simulink model "Microgrid_W"  (R2020a)
settings: Solver=ode15s  StartTime=0  StopTime=1440*1  MaxStep=1  RelTol=1e-3
libraries: simulink x4214, powerlib x685, simulink_extras x28, Microgrid_Library x18, powerlib_meascontrol x12
(part 4 of 48)

== system Microgrid_W/House 2 W3/Light 4 ==
  Add : Sum  Inputs=+++++++
  D1 : Subsystem
  D2 : Subsystem
  D3 : Subsystem
  D4 : Subsystem
  D5 : Subsystem
  D6 : Subsystem
  D7 : Subsystem
  Ground : powerlib/Elements/Ground  LConnTagsString=a
  Ideal Switch : powerlib/Power Electronics/Ideal Switch  Ron=V^2/(K_L3_W+0.000001)  Lon=0  IC=0  Rs=1e5  Cs=inf  Measurements=on
  + : PMIOPort  Side=Left
  wires:
  D7/1(Out1) -> Add/7
  D6/1(Out1) -> Add/6
  D5/1(Out1) -> Add/5
  D4/1(Out1) -> Add/4
  D3/1(Out1) -> Add/3
  D2/1(Out1) -> Add/2
  D1/1(Out1) -> Add/1
  Add/1 -> Ideal Switch/1
  connections:
  Ground/LConn1 -- Ideal Switch/LConn1
  +/RConn1 -- Ideal Switch/RConn1

== system Microgrid_W/House 2 W3/Light 5 ==
  Add : Sum  Inputs=+++++++
  D1 : Subsystem
  D2 : Subsystem
  D3 : Subsystem
  D4 : Subsystem
  D5 : Subsystem
  D6 : Subsystem
  D7 : Subsystem
  Ground : powerlib/Elements/Ground  LConnTagsString=a
  Ideal Switch : powerlib/Power Electronics/Ideal Switch  Ron=V^2/(K_L4_W+0.000001)  Lon=0  IC=0  Rs=1e5  Cs=inf  Measurements=on
  + : PMIOPort  Side=Left
  wires:
  D7/1(Out1) -> Add/7
  D6/1(Out1) -> Add/6
  D5/1(Out1) -> Add/5
  D4/1(Out1) -> Add/4
  D3/1(Out1) -> Add/3
  D2/1(Out1) -> Add/2
  D1/1(Out1) -> Add/1
  Add/1 -> Ideal Switch/1
  connections:
  Ground/LConn1 -- Ideal Switch/LConn1
  +/RConn1 -- Ideal Switch/RConn1

== system Microgrid_W/House 2 W3/Light 6 ==
  Add : Sum  Inputs=+++++++
  D1 : Subsystem
  D2 : Subsystem
  D3 : Subsystem
  D4 : Subsystem
  D5 : Subsystem
  D6 : Subsystem
  D7 : Subsystem
  Ground : powerlib/Elements/Ground  LConnTagsString=a
  Ideal Switch : powerlib/Power Electronics/Ideal Switch  Ron=V^2/(K_L5_W+0.000001)  Lon=0  IC=0  Rs=1e5  Cs=inf  Measurements=on
  + : PMIOPort  Side=Left
  wires:
  D1/1(Out1) -> Add/1
  D2/1(Out1) -> Add/2
  D3/1(Out1) -> Add/3
  D4/1(Out1) -> Add/4
  D5/1(Out1) -> Add/5
  D6/1(Out1) -> Add/6
  D7/1(Out1) -> Add/7
  Add/1 -> Ideal Switch/1
  connections:
  Ground/LConn1 -- Ideal Switch/LConn1
  +/RConn1 -- Ideal Switch/RConn1

== system Microgrid_W/House 2 W3/Light 7 ==
  Add : Sum  Inputs=+++++++
  D1 : Subsystem
  D2 : Subsystem
  D3 : Subsystem
  D4 : Subsystem
  D5 : Subsystem
  D6 : Subsystem
  D7 : Subsystem
  Ground : powerlib/Elements/Ground  LConnTagsString=a
  Ideal Switch : powerlib/Power Electronics/Ideal Switch  Ron=V^2/(K_L6_W+0.000001)  Lon=0  IC=0  Rs=1e5  Cs=inf  Measurements=on
  + : PMIOPort  Side=Left
  wires:
  D7/1(Out1) -> Add/7
  D6/1(Out1) -> Add/6
  D5/1(Out1) -> Add/5
  D4/1(Out1) -> Add/4
  D3/1(Out1) -> Add/3
  D2/1(Out1) -> Add/2
  D1/1(Out1) -> Add/1
  Add/1 -> Ideal Switch/1
  connections:
  Ground/LConn1 -- Ideal Switch/LConn1
  +/RConn1 -- Ideal Switch/RConn1

== system Microgrid_W/House 2 W3/Oven ==
  Add : Sum  Inputs=+++++++
  D1 : Subsystem
  D2 : Subsystem
  D3 : Subsystem
  D4 : Subsystem
  D5 : Subsystem
  D6 : Subsystem
  D7 : Subsystem
  Ground : powerlib/Elements/Ground  LConnTagsString=a
  Ideal Switch : powerlib/Power Electronics/Ideal Switch  Ron=V^2/(825*N_Elements+0.000001)  Lon=0  IC=0  Rs=1e5  Cs=inf  Measurements=on
  + : PMIOPort  Side=Left
  wires:
  D7/1(Out1) -> Add/7
  D6/1(Out1) -> Add/6
  D5/1(Out1) -> Add/5
  D4/1(Out1) -> Add/4
  D3/1(Out1) -> Add/3
  D2/1(Out1) -> Add/2
  D1/1(Out1) -> Add/1
  Add/1 -> Ideal Switch/1
  connections:
  +/RConn1 -- Ideal Switch/RConn1
  Ground/LConn1 -- Ideal Switch/LConn1

== system Microgrid_W/House 2 W3/Phone_Charger ==
  Add : Sum  Inputs=+++++++
  Add1 : Sum  Inputs=+++++++
  Add2 : Sum  Inputs=+++++++
  D1 : Subsystem
  D10 : Subsystem
  D11 : Subsystem
  D12 : Subsystem
  D13 : Subsystem
  D14 : Subsystem
  D15 : Subsystem
  D16 : Subsystem
  D17 : Subsystem
  D18 : Subsystem
  D19 : Subsystem
  D2 : Subsystem
  D20 : Subsystem
  D21 : Subsystem
  D3 : Subsystem
  D4 : Subsystem
  D5 : Subsystem
  D6 : Subsystem
  D7 : Subsystem
  D8 : Subsystem
  D9 : Subsystem
  Ground : powerlib/Elements/Ground  LConnTagsString=a
  Ideal Switch : powerlib/Power Electronics/Ideal Switch  Ron=V^2/(Phone_C_1_W+0.000001)  Lon=0  IC=0  Rs=1e5  Cs=inf  Measurements=on
  Ideal Switch1 : powerlib/Power Electronics/Ideal Switch  Ron=V^2/(Phone_C_2_W+0.000001)  Lon=0  IC=0  Rs=1e5  Cs=inf  Measurements=on
  Ideal Switch2 : powerlib/Power Electronics/Ideal Switch  Ron=V^2/(Phone_C_3_W+0.000001)  Lon=0  IC=0  Rs=1e5  Cs=inf  Measurements=on
  + : PMIOPort  Side=Left
  +1 : PMIOPort  Port=2  Side=Right
  +2 : PMIOPort  Port=3  Side=Left
  wires:
  D1/1(Out1) -> Add/1
  D2/1(Out1) -> Add/2
  D3/1(Out1) -> Add/3
  D4/1(Out1) -> Add/4
  D5/1(Out1) -> Add/5
  D6/1(Out1) -> Add/6
  D7/1(Out1) -> Add/7
  D8/1(Out1) -> Add1/1
  D9/1(Out1) -> Add1/2
  D10/1(Out1) -> Add1/3
  D11/1(Out1) -> Add1/4
  D12/1(Out1) -> Add1/5
  D13/1(Out1) -> Add1/6
  D14/1(Out1) -> Add1/7
  D20/1(Out1) -> Add2/1
  D15/1(Out1) -> Add2/2
  D16/1(Out1) -> Add2/3
  D17/1(Out1) -> Add2/4
  D18/1(Out1) -> Add2/5
  D19/1(Out1) -> Add2/6
  D21/1(Out1) -> Add2/7
  Add/1 -> Ideal Switch/1
  Add1/1 -> Ideal Switch1/1
  Add2/1 -> Ideal Switch2/1
  connections:
  Ground/LConn1 -- Ideal Switch2/LConn1 -- Ideal Switch1/LConn1 -- Ideal Switch/LConn1
  +/RConn1 -- Ideal Switch/RConn1
  +1/RConn1 -- Ideal Switch1/RConn1
  +2/RConn1 -- Ideal Switch2/RConn1

== system Microgrid_W/House 2 W3/Refrigerator ==
  Current Measurement : powerlib/Measurements/Current Measurement  PhasorSimulation=off  OutputType=Complex  PSBequivalent=0
  Ground : powerlib/Elements/Ground  LConnTagsString=a
  Ideal Switch : powerlib/Power Electronics/Ideal Switch  Ron=0.01  Lon=0  IC=0  Rs=1e5  Cs=inf  Measurements=on
  Ideal Switch1 : powerlib/Power Electronics/Ideal Switch  Ron=0.01  Lon=0  IC=0  Rs=1e5  Cs=inf  Measurements=on
  Monostable : powerlib_meascontrol/Logic/Monostable  EdgeDetect=Rising  PulseDuration=0.1*(60/t)  ic=0  Ts=0
      settings: SourceProductBaseCode=PS
  Product : Product
  Series RLC Branch1 : powerlib/Elements/Series RLC Branch  LConnTagsString=__new0  RConnTagsString=__new0  BranchType=R  Resistance=V^2/(2240-Fridge_W)  Inductance=1e-3  SetiL0=off  InitialCurrent=0  Capacitance=1e-6  Setx0=off  InitialVoltage=0  Measurements=None
  Series RLC Branch2 : powerlib/Elements/Series RLC Branch  LConnTagsString=__new0  RConnTagsString=__new0  BranchType=R  Resistance=V^2/Fridge_W  Inductance=1e-3  SetiL0=off  InitialCurrent=0  Capacitance=1e-6  Setx0=off  InitialVoltage=0  Measurements=None
  Subsystem : Subsystem
  Voltage Measurement : powerlib/Measurements/Voltage Measurement  PhasorSimulation=off  OutputType=Complex  PSBequivalent=0
  + : PMIOPort  Side=Left
  wires:
  Product/1 -> Subsystem/1(In1)
  Subsystem/1(Out1) -> Ideal Switch/1, Monostable/1
  Current Measurement/1 -> Product/1
  Voltage Measurement/1 -> Product/2
  Monostable/1 -> Ideal Switch1/1
  connections:
  Ground/LConn1 -- Voltage Measurement/LConn2 -- Series RLC Branch2/RConn1 -- Series RLC Branch1/RConn1
  Current Measurement/RConn1 -- Voltage Measurement/LConn1 -- Series RLC Branch2/LConn1
  +/RConn1 -- Ideal Switch/LConn1 -- Ideal Switch1/LConn1
  Ideal Switch/RConn1 -- Current Measurement/LConn1
  Series RLC Branch1/LConn1 -- Ideal Switch1/RConn1

== system Microgrid_W/House 2 W3/Shower ==
  Add : Sum  Inputs=+++++++
  D1 : Subsystem
  D2 : Subsystem
  D3 : Subsystem
  D4 : Subsystem
  D5 : Subsystem
  D6 : Subsystem
  D7 : Subsystem
  Divide : Product  Inputs=*/
  Gain : Gain  Gain=1/(60*(60/t))
  Mo : Constant  Value=9
  Product : Product
  Product1 : Product
  Subtract : Sum  Inputs=+-
  Subtract1 : Sum  Inputs=+-
  Tc : Constant  Value=7
  Th : Constant  Value=60
  To : Constant  Value=40
  Out1 : Outport  VectorParamsAs1DForOutWhenUnconnected=off
  wires:
  Tc/1 -> Subtract1/1, Subtract/1
  To/1 -> Subtract/2
  Th/1 -> Subtract1/2
  Subtract1/1 -> Divide/2
  Subtract/1 -> Product/2
  Mo/1 -> Product/1
  Product/1 -> Divide/1
  Product1/1 -> Gain/1
  Gain/1 -> Out1/1
  Divide/1 -> Product1/1
  D7/1(Out1) -> Add/7
  D6/1(Out1) -> Add/6
  D5/1(Out1) -> Add/5
  D4/1(Out1) -> Add/4
  D3/1(Out1) -> Add/3
  D2/1(Out1) -> Add/2
  D1/1(Out1) -> Add/1
  Add/1 -> Product1/2

== system Microgrid_W/House 2 W3/Stereo ==
  Add : Sum  Inputs=+++++++
  D1 : Subsystem
  D2 : Subsystem
  D3 : Subsystem
  D4 : Subsystem
  D5 : Subsystem
  D6 : Subsystem
  D7 : Subsystem
  Ground : powerlib/Elements/Ground  LConnTagsString=a
  Ideal Switch : powerlib/Power Electronics/Ideal Switch  Ron=V^2/((Stereo_W/2)*1.7+0.000001)+V^2/(Stereo_W/2)/2.2  Lon=0  IC=0  Rs=1e5  Cs=inf  Measurements=on
  + : PMIOPort  Side=Left
  wires:
  D7/1(Out1) -> Add/7
  D6/1(Out1) -> Add/6
  D5/1(Out1) -> Add/5
  D4/1(Out1) -> Add/4
  D3/1(Out1) -> Add/3
  D2/1(Out1) -> Add/2
  D1/1(Out1) -> Add/1
  Add/1 -> Ideal Switch/1
  connections:
  Ground/LConn1 -- Ideal Switch/LConn1
  +/RConn1 -- Ideal Switch/RConn1

== system Microgrid_W/House 2 W3/Subsystem ==

== system Microgrid_W/House 2 W3/Subsystem1 ==

== system Microgrid_W/House 2 W3/Subsystem2 ==

== system Microgrid_W/House 2 W3/Subsystem3 ==

== system Microgrid_W/House 2 W3/Subsystem4 ==

== system Microgrid_W/House 2 W3/Thermostat ==
  In1 : Inport
  Compare To Constant : simulink/Logic and Bit Operations/Compare To Constant  relop=>=  const=65  OutDataTypeStr=boolean
  Compare To Constant1 : simulink/Logic and Bit Operations/Compare To Constant  relop=<=  const=40  OutDataTypeStr=boolean
  Constant : Constant  Value=0
  Constant1 : Constant
  S-R Flip-Flop : simulink_extras/Flip Flops/S-R Flip-Flop  initial_condition=0
  Switch : Switch  Criteria=u2 > Threshold  Threshold=0.5
  Out1 : Outport  VectorParamsAs1DForOutWhenUnconnected=off
  wires:
  In1/1 -> Compare To Constant1/1, Compare To Constant/1
  Compare To Constant/1 -> S-R Flip-Flop/2
  Compare To Constant1/1 -> S-R Flip-Flop/1
  S-R Flip-Flop/1 -> Switch/2
  Switch/1 -> Out1/1
  Constant1/1 -> Switch/1
  Constant/1 -> Switch/3

== system Microgrid_W/House 2 W3/Toaster ==
  Add : Sum  Inputs=+++++++
  D1 : Subsystem
  D2 : Subsystem
  D3 : Subsystem
  D4 : Subsystem
  D5 : Subsystem
  D6 : Subsystem
  D7 : Subsystem
  Ground : powerlib/Elements/Ground  LConnTagsString=a
  Ideal Switch : powerlib/Power Electronics/Ideal Switch  Ron=V^2/(Toaster_W+0.000001)  Lon=0  IC=0  Rs=1e5  Cs=inf  Measurements=on
  + : PMIOPort  Side=Left
  wires:
  D7/1(Out1) -> Add/7
  D6/1(Out1) -> Add/6
  D5/1(Out1) -> Add/5
  D4/1(Out1) -> Add/4
  D3/1(Out1) -> Add/3
  D2/1(Out1) -> Add/2
  D1/1(Out1) -> Add/1
  Add/1 -> Ideal Switch/1
  connections:
  +/RConn1 -- Ideal Switch/RConn1
  Ground/LConn1 -- Ideal Switch/LConn1

== system Microgrid_W/House 2 W3/Tv ==
  Add : Sum  Inputs=+++++++
  D1 : Subsystem
  D2 : Subsystem
  D3 : Subsystem
  D4 : Subsystem
  D5 : Subsystem
  D6 : Subsystem
  D7 : Subsystem
  Ground : powerlib/Elements/Ground  LConnTagsString=a
  Ideal Switch : powerlib/Power Electronics/Ideal Switch  Ron=(V^2/(TV_W/2.85)*2.4+0.000001)+(V^2/(TV_W/2.64))  Lon=0  IC=0  Rs=1e5  Cs=inf  Measurements=on
  + : PMIOPort  Side=Left
  wires:
  D1/1(Out1) -> Add/1
  D2/1(Out1) -> Add/2
  D3/1(Out1) -> Add/3
  D4/1(Out1) -> Add/4
  D5/1(Out1) -> Add/5
  D6/1(Out1) -> Add/6
  D7/1(Out1) -> Add/7
  Add/1 -> Ideal Switch/1
  connections:
  Ground/LConn1 -- Ideal Switch/LConn1
  +/RConn1 -- Ideal Switch/RConn1

== system Microgrid_W/House 2 W3/Water tank ==
  Mass flow rate : Inport
  Add : Sum
  Add1 : Sum
  Constant : Constant
  Current Measurement : powerlib/Measurements/Current Measurement  PhasorSimulation=off  OutputType=Complex  PSBequivalent=0
  Divide : Product  Inputs=*/
  Divide1 : Product  Inputs=*/
  Gain : Gain  Gain=t
  Ground : powerlib/Elements/Ground  LConnTagsString=a
  Ideal Switch : powerlib/Power Electronics/Ideal Switch  Ron=V^2/HW_W  Lon=0  IC=0  Rs=1e5  Cs=inf  Measurements=on
  Integrator : Integrator
  Product1 : Product  Inputs=3
  Product2 : Product  Inputs=3
  Product3 : Product  Inputs=3
  Product4 : Product  Inputs=4
  Product5 : Product
  Product6 : Product
  Subtract : Sum  Inputs=++-
  Subtract1 : Sum  Inputs=+-
  Subtract2 : Sum  Inputs=+-
  Thermostat : Subsystem
  Ti : Constant  Value=Ti
  Ti1 : Constant  Value=4179
  Ti10 : Constant  Value=M
  Ti11 : Constant  Value=4179
  Ti12 : Constant  Value=60/t
  Ti2 : Constant  Value=1.5
  Ti3 : Constant  Value=Ta
  Ti4 : Constant  Value=pi
  Ti5 : Constant  Value=D
  Ti6 : Constant  Value=L
  Ti7 : Constant  Value=D
  Ti8 : Constant  Value=2
  Ti9 : Constant  Value=pi
  Voltage Measurement : powerlib/Measurements/Voltage Measurement  PhasorSimulation=off  OutputType=Complex  PSBequivalent=0
  + : PMIOPort  Side=Left
  Temperature : Outport
  wires:
  Constant/1 -> Ideal Switch/1
  Subtract1/1 -> Product1/1
  Product1/1 -> Subtract/2
  Product6/1 -> Subtract/1
  Ti/1 -> Subtract1/1
  Mass flow rate/1 -> Product1/2
  Ti1/1 -> Product1/3
  Product2/1 -> Subtract/3
  Ti2/1 -> Product2/1
  Add/1 -> Product2/2
  Subtract2/1 -> Product2/3
  Ti3/1 -> Subtract2/2
  Product3/1 -> Add/1
  Product4/1 -> Add/2
  Ti5/1 -> Product3/2
  Ti4/1 -> Product3/1
  Ti6/1 -> Product3/3
  Divide/1 -> Product4/1, Product4/2
  Ti7/1 -> Divide/1
  Ti8/1 -> Product4/3, Divide/2
  Ti9/1 -> Product4/4
  Ti10/1 -> Product5/1
  Ti11/1 -> Product5/2
  Product5/1 -> Divide1/2
  Subtract/1 -> Divide1/1
  Divide1/1 -> Integrator/1
  Integrator/1 -> Add1/2
  Ti12/1 -> Add1/1
  Add1/1 -> Gain/1
  Gain/1 -> Subtract1/2, Subtract2/1, Thermostat/1(In1), Temperature/1
  Current Measurement/1 -> Product6/1
  Voltage Measurement/1 -> Product6/2
  connections:
  Current Measurement/RConn1 -- Voltage Measurement/LConn1 -- Ideal Switch/RConn1
  Current Measurement/LConn1 -- +/RConn1
  Ground/LConn1 -- Voltage Measurement/LConn2 -- Ideal Switch/LConn1

== system Microgrid_W/House 3 W1/Clock 1 ==
  Ground : powerlib/Elements/Ground  LConnTagsString=a
  Series RLC Branch2 : powerlib/Elements/Series RLC Branch  LConnTagsString=__new0  RConnTagsString=__new0  BranchType=R  Resistance=V^2/(Clock_1_W+0.000001)  Inductance=1e-3  SetiL0=off  InitialCurrent=0  Capacitance=1e-6  Setx0=off  InitialVoltage=0  Measurements=None
  + : PMIOPort  Side=Left
  connections:
  Ground/LConn1 -- Series RLC Branch2/RConn1
  +/RConn1 -- Series RLC Branch2/LConn1

== system Microgrid_W/House 3 W1/Clock 2 ==
  Ground : powerlib/Elements/Ground  LConnTagsString=a
  Series RLC Branch2 : powerlib/Elements/Series RLC Branch  LConnTagsString=__new0  RConnTagsString=__new0  BranchType=R  Resistance=V^2/(Clock_2_W+0.000001)  Inductance=1e-3  SetiL0=off  InitialCurrent=0  Capacitance=1e-6  Setx0=off  InitialVoltage=0  Measurements=None
  + : PMIOPort  Side=Left
  connections:
  Ground/LConn1 -- Series RLC Branch2/RConn1
  +/RConn1 -- Series RLC Branch2/LConn1

== system Microgrid_W/House 3 W1/Heater ==
  Add : Sum  Inputs=+++++++
  D1 : Subsystem
  D2 : Subsystem
  D3 : Subsystem
  D4 : Subsystem
  D5 : Subsystem
  D6 : Subsystem
  D7 : Subsystem
  Ground : powerlib/Elements/Ground  LConnTagsString=a
  Ideal Switch : powerlib/Power Electronics/Ideal Switch  Ron=V^2/Heater_W  Lon=0  IC=0  Rs=1e5  Cs=inf  Measurements=on
  + : PMIOPort  Side=Left
  wires:
  Add/1 -> Ideal Switch/1
  D1/1(Out1) -> Add/1
  D2/1(Out1) -> Add/2
  D3/1(Out1) -> Add/3
  D4/1(Out1) -> Add/4
  D5/1(Out1) -> Add/5
  D6/1(Out1) -> Add/6
  D7/1(Out1) -> Add/7
  connections:
  Ground/LConn1 -- Ideal Switch/LConn1
  +/RConn1 -- Ideal Switch/RConn1

== system Microgrid_W/House 3 W1/Kettle ==
  Add : Sum  Inputs=+++++++
  D1 : Subsystem
  D2 : Subsystem
  D3 : Subsystem
  D4 : Subsystem
  D5 : Subsystem
  D6 : Subsystem
  D7 : Subsystem
  Ground : powerlib/Elements/Ground  LConnTagsString=a
  Ideal Switch : powerlib/Power Electronics/Ideal Switch  Ron=V^2/(Jug_W+0.000001)  Lon=0  IC=0  Rs=1e5  Cs=inf  Measurements=on
  + : PMIOPort  Side=Left
  wires:
  Add/1 -> Ideal Switch/1
  D1/1(Out1) -> Add/1
  D2/1(Out1) -> Add/2
  D3/1(Out1) -> Add/3
  D4/1(Out1) -> Add/4
  D5/1(Out1) -> Add/5
  D6/1(Out1) -> Add/6
  D7/1(Out1) -> Add/7
  connections:
  Ground/LConn1 -- Ideal Switch/LConn1
  +/RConn1 -- Ideal Switch/RConn1

== system Microgrid_W/House 3 W1/Lamp 1 ==
  Add : Sum  Inputs=+++++++
  D1 : Subsystem
  D2 : Subsystem
  D3 : Subsystem
  D4 : Subsystem
  D5 : Subsystem
  D6 : Subsystem
  D7 : Subsystem
  Ground : powerlib/Elements/Ground  LConnTagsString=a
  Ideal Switch : powerlib/Power Electronics/Ideal Switch  Ron=V^2/(Lamp_1_W+0.000001)  Lon=0  IC=0  Rs=1e5  Cs=inf  Measurements=on
  + : PMIOPort  Side=Left
  wires:
  Add/1 -> Ideal Switch/1
  D7/1(Out1) -> Add/7
  D6/1(Out1) -> Add/6
  D5/1(Out1) -> Add/5
  D4/1(Out1) -> Add/4
  D3/1(Out1) -> Add/3
  D2/1(Out1) -> Add/2
  D1/1(Out1) -> Add/1
  connections:
  +/RConn1 -- Ideal Switch/RConn1
  Ground/LConn1 -- Ideal Switch/LConn1

== system Microgrid_W/House 3 W1/Lamp 2 ==
  Add : Sum  Inputs=+++++++
  D1 : Subsystem
  D2 : Subsystem
  D3 : Subsystem
  D4 : Subsystem
  D5 : Subsystem
  D6 : Subsystem
  D7 : Subsystem
  Ground : powerlib/Elements/Ground  LConnTagsString=a
  Ideal Switch : powerlib/Power Electronics/Ideal Switch  Ron=V^2/(Lamp_2_W+0.000001)  Lon=0  IC=0  Rs=1e5  Cs=inf  Measurements=on
  + : PMIOPort  Side=Left
  wires:
  Add/1 -> Ideal Switch/1
  D1/1(Out1) -> Add/1
  D2/1(Out1) -> Add/2
  D3/1(Out1) -> Add/3
  D4/1(Out1) -> Add/4
  D5/1(Out1) -> Add/5
  D6/1(Out1) -> Add/6
  D7/1(Out1) -> Add/7
  connections:
  +/RConn1 -- Ideal Switch/RConn1
  Ground/LConn1 -- Ideal Switch/LConn1

== system Microgrid_W/House 3 W1/Lamp 3 ==
  Add : Sum  Inputs=+++++++
  D1 : Subsystem
  D2 : Subsystem
  D3 : Subsystem
  D4 : Subsystem
  D5 : Subsystem
  D6 : Subsystem
  D7 : Subsystem
  Ground : powerlib/Elements/Ground  LConnTagsString=a
  Ideal Switch : powerlib/Power Electronics/Ideal Switch  Ron=V^2/(Lamp_3_W+0.000001)  Lon=0  IC=0  Rs=1e5  Cs=inf  Measurements=on
  + : PMIOPort  Side=Left
  wires:
  Add/1 -> Ideal Switch/1
  D7/1(Out1) -> Add/7
  D6/1(Out1) -> Add/6
  D5/1(Out1) -> Add/5
  D4/1(Out1) -> Add/4
  D3/1(Out1) -> Add/3
  D2/1(Out1) -> Add/2
  D1/1(Out1) -> Add/1
  connections:
  +/RConn1 -- Ideal Switch/RConn1
  Ground/LConn1 -- Ideal Switch/LConn1

== system Microgrid_W/House 3 W1/Laptop_Charger ==
  Add : Sum  Inputs=+++++++
  Add1 : Sum  Inputs=+++++++
  D1 : Subsystem
  D10 : Subsystem
  D11 : Subsystem
  D12 : Subsystem
  D13 : Subsystem
  D14 : Subsystem
  D2 : Subsystem
  D3 : Subsystem
  D4 : Subsystem
  D5 : Subsystem
  D6 : Subsystem
  D7 : Subsystem
  D8 : Subsystem
  D9 : Subsystem
  Ground : powerlib/Elements/Ground  LConnTagsString=a
  Ground1 : powerlib/Elements/Ground  LConnTagsString=a
  Ideal Switch : powerlib/Power Electronics/Ideal Switch  Ron=V^2/(Laptop_C_1_W+0.000001)  Lon=0  IC=0  Rs=1e5  Cs=inf  Measurements=on
  Ideal Switch1 : powerlib/Power Electronics/Ideal Switch  Ron=V^2/(Laptop_C_2_W+0.000001)  Lon=0  IC=0  Rs=1e5  Cs=inf  Measurements=on
  + : PMIOPort  Side=Left
  +1 : PMIOPort  Port=2  Side=Right
  wires:
  Add/1 -> Ideal Switch1/1
  Add1/1 -> Ideal Switch/1
  D8/1(Out1) -> Add1/1
  D9/1(Out1) -> Add1/2
  D10/1(Out1) -> Add1/3
  D11/1(Out1) -> Add1/4
  D12/1(Out1) -> Add1/5
  D13/1(Out1) -> Add1/6
  D14/1(Out1) -> Add1/7
  D7/1(Out1) -> Add/7
  D6/1(Out1) -> Add/6
  D5/1(Out1) -> Add/5
  D4/1(Out1) -> Add/4
  D3/1(Out1) -> Add/3
  D2/1(Out1) -> Add/2
  D1/1(Out1) -> Add/1
  connections:
  +1/RConn1 -- Ideal Switch1/RConn1
  Ground1/LConn1 -- Ideal Switch1/LConn1
  +/RConn1 -- Ideal Switch/RConn1
  Ground/LConn1 -- Ideal Switch/LConn1

== system Microgrid_W/House 3 W1/Light 1 ==
  Add : Sum  Inputs=+++++++
  D1 : Subsystem
  D2 : Subsystem
  D3 : Subsystem
  D4 : Subsystem
  D5 : Subsystem
  D6 : Subsystem
  D7 : Subsystem
  Ground : powerlib/Elements/Ground  LConnTagsString=a
  Ideal Switch : powerlib/Power Electronics/Ideal Switch  Ron=V^2/(K_L1_W + 0.000001)  Lon=0  IC=0  Rs=1e5  Cs=inf  Measurements=on
  + : PMIOPort  Side=Left
  wires:
  D7/1(Out1) -> Add/7
  D6/1(Out1) -> Add/6
  D5/1(Out1) -> Add/5
  D4/1(Out1) -> Add/4
  D3/1(Out1) -> Add/3
  D2/1(Out1) -> Add/2
  D1/1(Out1) -> Add/1
  Add/1 -> Ideal Switch/1
  connections:
  Ground/LConn1 -- Ideal Switch/LConn1
  +/RConn1 -- Ideal Switch/RConn1

== system Microgrid_W/House 3 W1/Light 2 ==
  Add : Sum  Inputs=+++++++
  D1 : Subsystem
  D2 : Subsystem
  D3 : Subsystem
  D4 : Subsystem
  D5 : Subsystem
  D6 : Subsystem
  D7 : Subsystem
  Ground : powerlib/Elements/Ground  LConnTagsString=a
  Ideal Switch : powerlib/Power Electronics/Ideal Switch  Ron=V^2/(K_L2_W+0.000001)  Lon=0  IC=0  Rs=1e5  Cs=inf  Measurements=on
  + : PMIOPort  Side=Left
  wires:
  Add/1 -> Ideal Switch/1
  D1/1(Out1) -> Add/1
  D2/1(Out1) -> Add/2
  D3/1(Out1) -> Add/3
  D4/1(Out1) -> Add/4
  D5/1(Out1) -> Add/5
  D6/1(Out1) -> Add/6
  D7/1(Out1) -> Add/7
  connections:
  Ground/LConn1 -- Ideal Switch/LConn1
  +/RConn1 -- Ideal Switch/RConn1

== system Microgrid_W/House 3 W1/Light 3 ==
  Add : Sum  Inputs=+++++++
  D1 : Subsystem
  D2 : Subsystem
  D3 : Subsystem
  D4 : Subsystem
  D5 : Subsystem
  D6 : Subsystem
  D7 : Subsystem
  Ground : powerlib/Elements/Ground  LConnTagsString=a
  Ideal Switch : powerlib/Power Electronics/Ideal Switch  Ron=V^2/(K_L3_W+0.000001)  Lon=0  IC=0  Rs=1e5  Cs=inf  Measurements=on
  + : PMIOPort  Side=Left
  wires:
  Add/1 -> Ideal Switch/1
  D1/1(Out1) -> Add/1
  D2/1(Out1) -> Add/2
  D3/1(Out1) -> Add/3
  D4/1(Out1) -> Add/4
  D5/1(Out1) -> Add/5
  D6/1(Out1) -> Add/6
  D7/1(Out1) -> Add/7
  connections:
  +/RConn1 -- Ideal Switch/RConn1
  Ground/LConn1 -- Ideal Switch/LConn1

== system Microgrid_W/House 3 W1/Light 4 ==
  Add : Sum  Inputs=+++++++
  D1 : Subsystem
  D2 : Subsystem
  D3 : Subsystem
  D4 : Subsystem
  D5 : Subsystem
  D6 : Subsystem
  D7 : Subsystem
  Ground : powerlib/Elements/Ground  LConnTagsString=a
  Ideal Switch : powerlib/Power Electronics/Ideal Switch  Ron=V^2/(K_L4_W+0.000001)  Lon=0  IC=0  Rs=1e5  Cs=inf  Measurements=on
  + : PMIOPort  Side=Left
  wires:
  Add/1 -> Ideal Switch/1
  D1/1(Out1) -> Add/1
  D2/1(Out1) -> Add/2
  D3/1(Out1) -> Add/3
  D4/1(Out1) -> Add/4
  D5/1(Out1) -> Add/5
  D6/1(Out1) -> Add/6
  D7/1(Out1) -> Add/7
  connections:
  +/RConn1 -- Ideal Switch/RConn1
  Ground/LConn1 -- Ideal Switch/LConn1

== system Microgrid_W/House 3 W1/Light 5 ==
  Add : Sum  Inputs=+++++++
  D1 : Subsystem
  D2 : Subsystem
  D3 : Subsystem
  D4 : Subsystem
  D5 : Subsystem
  D6 : Subsystem
  D7 : Subsystem
  Ground : powerlib/Elements/Ground  LConnTagsString=a
  Ideal Switch : powerlib/Power Electronics/Ideal Switch  Ron=V^2/(K_L5_W+0.000001)  Lon=0  IC=0  Rs=1e5  Cs=inf  Measurements=on
  + : PMIOPort  Side=Left
  wires:
  Add/1 -> Ideal Switch/1
  D7/1(Out1) -> Add/7
  D6/1(Out1) -> Add/6
  D5/1(Out1) -> Add/5
  D4/1(Out1) -> Add/4
  D3/1(Out1) -> Add/3
  D2/1(Out1) -> Add/2
  D1/1(Out1) -> Add/1
  connections:
  +/RConn1 -- Ideal Switch/RConn1
  Ground/LConn1 -- Ideal Switch/LConn1

== system Microgrid_W/House 3 W1/Light 6 ==
  Add : Sum  Inputs=+++++++
  D1 : Subsystem
  D2 : Subsystem
  D3 : Subsystem
  D4 : Subsystem
  D5 : Subsystem
  D6 : Subsystem
  D7 : Subsystem
  Ground : powerlib/Elements/Ground  LConnTagsString=a
  Ideal Switch : powerlib/Power Electronics/Ideal Switch  Ron=V^2/(K_L6_W+0.000001)  Lon=0  IC=0  Rs=1e5  Cs=inf  Measurements=on
  + : PMIOPort  Side=Left
  wires:
  Add/1 -> Ideal Switch/1
  D1/1(Out1) -> Add/1
  D2/1(Out1) -> Add/2
  D3/1(Out1) -> Add/3
  D4/1(Out1) -> Add/4
  D5/1(Out1) -> Add/5
  D6/1(Out1) -> Add/6
  D7/1(Out1) -> Add/7
  connections:
  +/RConn1 -- Ideal Switch/RConn1
  Ground/LConn1 -- Ideal Switch/LConn1

== system Microgrid_W/House 3 W1/Oven ==
  Add : Sum  Inputs=+++++++
  D1 : Subsystem
  D2 : Subsystem
  D3 : Subsystem
  D4 : Subsystem
  D5 : Subsystem
  D6 : Subsystem
  D7 : Subsystem
  Ground : powerlib/Elements/Ground  LConnTagsString=a
  Ideal Switch : powerlib/Power Electronics/Ideal Switch  Ron=V^2/(825*N_Elements+0.000001)  Lon=0  IC=0  Rs=1e5  Cs=inf  Measurements=on
  + : PMIOPort  Side=Left
  wires:
  Add/1 -> Ideal Switch/1
  D1/1(Out1) -> Add/1
  D2/1(Out1) -> Add/2
  D3/1(Out1) -> Add/3
  D4/1(Out1) -> Add/4
  D5/1(Out1) -> Add/5
  D6/1(Out1) -> Add/6
  D7/1(Out1) -> Add/7
  connections:
  Ground/LConn1 -- Ideal Switch/LConn1
  +/RConn1 -- Ideal Switch/RConn1

== system Microgrid_W/House 3 W1/Phone_Charger ==
  Add : Sum  Inputs=+++++++
  Add1 : Sum  Inputs=+++++++
  Add2 : Sum  Inputs=+++++++
  D1 : Subsystem
  D10 : Subsystem
  D11 : Subsystem
  D12 : Subsystem
  D13 : Subsystem
  D14 : Subsystem
  D15 : Subsystem
  D16 : Subsystem
  D17 : Subsystem
  D18 : Subsystem
  D19 : Subsystem
  D2 : Subsystem
  D20 : Subsystem
  D21 : Subsystem
  D3 : Subsystem
  D4 : Subsystem
  D5 : Subsystem
  D6 : Subsystem
  D7 : Subsystem
  D8 : Subsystem
  D9 : Subsystem
  Ground : powerlib/Elements/Ground  LConnTagsString=a
  Ideal Switch : powerlib/Power Electronics/Ideal Switch  Ron=V^2/(Phone_C_1_W+0.000001)  Lon=0  IC=0  Rs=1e5  Cs=inf  Measurements=on
  Ideal Switch1 : powerlib/Power Electronics/Ideal Switch  Ron=V^2/(Phone_C_2_W+0.000001)  Lon=0  IC=0  Rs=1e5  Cs=inf  Measurements=on
  Ideal Switch2 : powerlib/Power Electronics/Ideal Switch  Ron=V^2/(Phone_C_3_W+0.000001)  Lon=0  IC=0  Rs=1e5  Cs=inf  Measurements=on
  + : PMIOPort  Side=Left
  +1 : PMIOPort  Port=2  Side=Right
  +2 : PMIOPort  Port=3  Side=Left
  wires:
  Add2/1 -> Ideal Switch2/1
  Add1/1 -> Ideal Switch1/1
  Add/1 -> Ideal Switch/1
  D21/1(Out1) -> Add2/7
  D19/1(Out1) -> Add2/6
  D18/1(Out1) -> Add2/5
  D17/1(Out1) -> Add2/4
  D16/1(Out1) -> Add2/3
  D15/1(Out1) -> Add2/2
  D20/1(Out1) -> Add2/1
  D14/1(Out1) -> Add1/7
  D13/1(Out1) -> Add1/6
  D12/1(Out1) -> Add1/5
  D11/1(Out1) -> Add1/4
  D10/1(Out1) -> Add1/3
  D9/1(Out1) -> Add1/2
  D8/1(Out1) -> Add1/1
  D7/1(Out1) -> Add/7
  D6/1(Out1) -> Add/6
  D5/1(Out1) -> Add/5
  D4/1(Out1) -> Add/4
  D3/1(Out1) -> Add/3
  D2/1(Out1) -> Add/2
  D1/1(Out1) -> Add/1
  connections:
  +2/RConn1 -- Ideal Switch2/RConn1
  +1/RConn1 -- Ideal Switch1/RConn1
  +/RConn1 -- Ideal Switch/RConn1
  Ideal Switch/LConn1 -- Ideal Switch1/LConn1 -- Ideal Switch2/LConn1 -- Ground/LConn1

== system Microgrid_W/House 3 W1/Refrigerator ==
  Current Measurement : powerlib/Measurements/Current Measurement  PhasorSimulation=off  OutputType=Complex  PSBequivalent=0
  Ground : powerlib/Elements/Ground  LConnTagsString=a
  Ideal Switch : powerlib/Power Electronics/Ideal Switch  Ron=0.01  Lon=0  IC=0  Rs=1e5  Cs=inf  Measurements=on
  Ideal Switch1 : powerlib/Power Electronics/Ideal Switch  Ron=0.01  Lon=0  IC=0  Rs=1e5  Cs=inf  Measurements=on
  Monostable : powerlib_meascontrol/Logic/Monostable  EdgeDetect=Rising  PulseDuration=0.1*(60/t)  ic=0  Ts=0
      settings: SourceProductBaseCode=PS
  Product : Product
  Series RLC Branch1 : powerlib/Elements/Series RLC Branch  LConnTagsString=__new0  RConnTagsString=__new0  BranchType=R  Resistance=V^2/(2240-Fridge_W)  Inductance=1e-3  SetiL0=off  InitialCurrent=0  Capacitance=1e-6  Setx0=off  InitialVoltage=0  Measurements=None
  Series RLC Branch2 : powerlib/Elements/Series RLC Branch  LConnTagsString=__new0  RConnTagsString=__new0  BranchType=R  Resistance=V^2/Fridge_W  Inductance=1e-3  SetiL0=off  InitialCurrent=0  Capacitance=1e-6  Setx0=off  InitialVoltage=0  Measurements=None
  Subsystem : Subsystem
  Voltage Measurement : powerlib/Measurements/Voltage Measurement  PhasorSimulation=off  OutputType=Complex  PSBequivalent=0
  + : PMIOPort  Side=Left
  wires:
  Monostable/1 -> Ideal Switch1/1
  Voltage Measurement/1 -> Product/2
  Current Measurement/1 -> Product/1
  Subsystem/1(Out1) -> Monostable/1, Ideal Switch/1
  Product/1 -> Subsystem/1(In1)
  connections:
  Series RLC Branch1/LConn1 -- Ideal Switch1/RConn1
  Ideal Switch/RConn1 -- Current Measurement/LConn1
  +/RConn1 -- Ideal Switch1/LConn1 -- Ideal Switch/LConn1
  Series RLC Branch2/LConn1 -- Voltage Measurement/LConn1 -- Current Measurement/RConn1
  Ground/LConn1 -- Series RLC Branch1/RConn1 -- Series RLC Branch2/RConn1 -- Voltage Measurement/LConn2

== system Microgrid_W/House 3 W1/Shower ==
  Add : Sum  Inputs=+++++++
  D1 : Subsystem
  D2 : Subsystem
  D3 : Subsystem
  D4 : Subsystem
  D5 : Subsystem
  D6 : Subsystem
  D7 : Subsystem
  Divide : Product  Inputs=*/
  Gain : Gain  Gain=1/(60*(60/t))
  Mo : Constant  Value=9
  Product : Product
  Product1 : Product
  Subtract : Sum  Inputs=+-
  Subtract1 : Sum  Inputs=+-
  Tc : Constant  Value=7
  Th : Constant  Value=60
  To : Constant  Value=40
  Out1 : Outport  VectorParamsAs1DForOutWhenUnconnected=off
  wires:
  Add/1 -> Product1/2
  D1/1(Out1) -> Add/1
  D2/1(Out1) -> Add/2
  D3/1(Out1) -> Add/3
  D4/1(Out1) -> Add/4
  D5/1(Out1) -> Add/5
  D6/1(Out1) -> Add/6
  D7/1(Out1) -> Add/7
  Divide/1 -> Product1/1
  Gain/1 -> Out1/1
  Product1/1 -> Gain/1
  Product/1 -> Divide/1
  Mo/1 -> Product/1
  Subtract/1 -> Product/2
  Subtract1/1 -> Divide/2
  Th/1 -> Subtract1/2
  To/1 -> Subtract/2
  Tc/1 -> Subtract/1, Subtract1/1

== system Microgrid_W/House 3 W1/Stereo ==
  Add : Sum  Inputs=+++++++
  D1 : Subsystem
  D2 : Subsystem
  D3 : Subsystem
  D4 : Subsystem
  D5 : Subsystem
  D6 : Subsystem
  D7 : Subsystem
  Ground : powerlib/Elements/Ground  LConnTagsString=a
  Ideal Switch : powerlib/Power Electronics/Ideal Switch  Ron=V^2/((Stereo_W/2)*1.7+0.000001)+V^2/(Stereo_W/2)/2.2  Lon=0  IC=0  Rs=1e5  Cs=inf  Measurements=on
  + : PMIOPort  Side=Left
  wires:
  Add/1 -> Ideal Switch/1
  D1/1(Out1) -> Add/1
  D2/1(Out1) -> Add/2
  D3/1(Out1) -> Add/3
  D4/1(Out1) -> Add/4
  D5/1(Out1) -> Add/5
  D6/1(Out1) -> Add/6
  D7/1(Out1) -> Add/7
  connections:
  +/RConn1 -- Ideal Switch/RConn1
  Ground/LConn1 -- Ideal Switch/LConn1

== system Microgrid_W/House 3 W1/Subsystem ==

== system Microgrid_W/House 3 W1/Subsystem1 ==

== system Microgrid_W/House 3 W1/Subsystem2 ==

== system Microgrid_W/House 3 W1/Subsystem3 ==

== system Microgrid_W/House 3 W1/Subsystem4 ==

== system Microgrid_W/House 3 W1/Toaster ==
  Add : Sum  Inputs=+++++++
  D1 : Subsystem
  D2 : Subsystem
  D3 : Subsystem
  D4 : Subsystem
  D5 : Subsystem
  D6 : Subsystem
  D7 : Subsystem
  Ground : powerlib/Elements/Ground  LConnTagsString=a
  Ideal Switch : powerlib/Power Electronics/Ideal Switch  Ron=V^2/(Toaster_W+0.000001)  Lon=0  IC=0  Rs=1e5  Cs=inf  Measurements=on
  + : PMIOPort  Side=Left
  wires:
  Add/1 -> Ideal Switch/1
  D1/1(Out1) -> Add/1
  D2/1(Out1) -> Add/2
  D3/1(Out1) -> Add/3
  D4/1(Out1) -> Add/4
  D5/1(Out1) -> Add/5
  D6/1(Out1) -> Add/6
  D7/1(Out1) -> Add/7
  connections:
  Ground/LConn1 -- Ideal Switch/LConn1
  +/RConn1 -- Ideal Switch/RConn1

== system Microgrid_W/House 3 W1/Tv ==
  Add : Sum  Inputs=+++++++
  D1 : Subsystem
  D2 : Subsystem
  D3 : Subsystem
  D4 : Subsystem
  D5 : Subsystem
  D6 : Subsystem
  D7 : Subsystem
  Ground : powerlib/Elements/Ground  LConnTagsString=a
  Ideal Switch : powerlib/Power Electronics/Ideal Switch  Ron=(V^2/(TV_W/2.85)*2.4+0.000001)+(V^2/(TV_W/2.64))  Lon=0  IC=0  Rs=1e5  Cs=inf  Measurements=on
  + : PMIOPort  Side=Left
  wires:
  Add/1 -> Ideal Switch/1
  D7/1(Out1) -> Add/7
  D6/1(Out1) -> Add/6
  D5/1(Out1) -> Add/5
  D4/1(Out1) -> Add/4
  D3/1(Out1) -> Add/3
  D2/1(Out1) -> Add/2
  D1/1(Out1) -> Add/1
  connections:
  +/RConn1 -- Ideal Switch/RConn1
  Ground/LConn1 -- Ideal Switch/LConn1

== system Microgrid_W/House 3 W1/Water tank ==
  Mass flow rate : Inport
  Add : Sum
  Add1 : Sum
  Current Measurement : powerlib/Measurements/Current Measurement  PhasorSimulation=off  OutputType=Complex  PSBequivalent=0
  Divide : Product  Inputs=*/
  Divide1 : Product  Inputs=*/
  Gain : Gain  Gain=t
  Ground : powerlib/Elements/Ground  LConnTagsString=a
  Ideal Switch : powerlib/Power Electronics/Ideal Switch  Ron=V^2/HW_W  Lon=0  IC=0  Rs=1e5  Cs=inf  Measurements=on
  Integrator : Integrator
  Product1 : Product  Inputs=3
  Product2 : Product  Inputs=3
  Product3 : Product  Inputs=3
  Product4 : Product  Inputs=4
  Product5 : Product
  Product6 : Product
  Subtract : Sum  Inputs=++-
  Subtract1 : Sum  Inputs=+-
  Subtract2 : Sum  Inputs=+-
  Thermostat : Subsystem
  Ti : Constant  Value=Ti
  Ti1 : Constant  Value=4179
  Ti10 : Constant  Value=M
  Ti11 : Constant  Value=4179
  Ti12 : Constant  Value=60/t
  Ti2 : Constant  Value=1.5
  Ti3 : Constant  Value=Ta
  Ti4 : Constant  Value=pi
  Ti5 : Constant  Value=D
  Ti6 : Constant  Value=L
  Ti7 : Constant  Value=D
  Ti8 : Constant  Value=2
  Ti9 : Constant  Value=pi
  Voltage Measurement : powerlib/Measurements/Voltage Measurement  PhasorSimulation=off  OutputType=Complex  PSBequivalent=0
  + : PMIOPort  Side=Left
  Temperature : Outport
  wires:
  Voltage Measurement/1 -> Product6/2
  Current Measurement/1 -> Product6/1
  Gain/1 -> Temperature/1, Subtract2/1, Subtract1/2, Thermostat/1(In1)
  Add1/1 -> Gain/1
  Ti12/1 -> Add1/1
  Integrator/1 -> Add1/2
  Divide1/1 -> Integrator/1
  Subtract/1 -> Divide1/1
  Product5/1 -> Divide1/2
  Ti11/1 -> Product5/2
  Ti10/1 -> Product5/1
  Ti9/1 -> Product4/4
  Ti8/1 -> Divide/2, Product4/3
  Ti7/1 -> Divide/1
  Divide/1 -> Product4/2, Product4/1
  Ti6/1 -> Product3/3
  Ti4/1 -> Product3/1
  Ti5/1 -> Product3/2
  Product4/1 -> Add/2
  Product3/1 -> Add/1
  Ti3/1 -> Subtract2/2
  Subtract2/1 -> Product2/3
  Add/1 -> Product2/2
  Ti2/1 -> Product2/1
  Product2/1 -> Subtract/3
  Ti1/1 -> Product1/3
  Mass flow rate/1 -> Product1/2
  Ti/1 -> Subtract1/1
  Product6/1 -> Subtract/1
  Product1/1 -> Subtract/2
  Subtract1/1 -> Product1/1
  Thermostat/1(Out1) -> Ideal Switch/1
  connections:
  Ideal Switch/LConn1 -- Voltage Measurement/LConn2 -- Ground/LConn1
  Current Measurement/LConn1 -- +/RConn1
  Ideal Switch/RConn1 -- Voltage Measurement/LConn1 -- Current Measurement/RConn1

== system Microgrid_W/House 3 W2/Clock 1 ==
  Ground : powerlib/Elements/Ground  LConnTagsString=a
  Series RLC Branch2 : powerlib/Elements/Series RLC Branch  LConnTagsString=__new0  RConnTagsString=__new0  BranchType=R  Resistance=V^2/(Clock_1_W+0.000001)  Inductance=1e-3  SetiL0=off  InitialCurrent=0  Capacitance=1e-6  Setx0=off  InitialVoltage=0  Measurements=None
  + : PMIOPort  Side=Left
  connections:
  Ground/LConn1 -- Series RLC Branch2/RConn1
  +/RConn1 -- Series RLC Branch2/LConn1

== system Microgrid_W/House 3 W2/Clock 2 ==
  Ground : powerlib/Elements/Ground  LConnTagsString=a
  Series RLC Branch2 : powerlib/Elements/Series RLC Branch  LConnTagsString=__new0  RConnTagsString=__new0  BranchType=R  Resistance=V^2/(Clock_2_W+0.000001)  Inductance=1e-3  SetiL0=off  InitialCurrent=0  Capacitance=1e-6  Setx0=off  InitialVoltage=0  Measurements=None
  + : PMIOPort  Side=Left
  connections:
  Ground/LConn1 -- Series RLC Branch2/RConn1
  +/RConn1 -- Series RLC Branch2/LConn1

== system Microgrid_W/House 3 W2/Heater ==
  Add : Sum  Inputs=+++++++
  D1 : Subsystem
  D2 : Subsystem
  D3 : Subsystem
  D4 : Subsystem
  D5 : Subsystem
  D6 : Subsystem
  D7 : Subsystem
  Ground : powerlib/Elements/Ground  LConnTagsString=a
  Ideal Switch : powerlib/Power Electronics/Ideal Switch  Ron=V^2/Heater_W  Lon=0  IC=0  Rs=1e5  Cs=inf  Measurements=on
  + : PMIOPort  Side=Left
  wires:
  Add/1 -> Ideal Switch/1
  D1/1(Out1) -> Add/1
  D2/1(Out1) -> Add/2
  D3/1(Out1) -> Add/3
  D4/1(Out1) -> Add/4
  D5/1(Out1) -> Add/5
  D6/1(Out1) -> Add/6
  D7/1(Out1) -> Add/7
  connections:
  Ground/LConn1 -- Ideal Switch/LConn1
  +/RConn1 -- Ideal Switch/RConn1

== system Microgrid_W/House 3 W2/Kettle ==
  Add : Sum  Inputs=+++++++
  D1 : Subsystem
  D2 : Subsystem
  D3 : Subsystem
  D4 : Subsystem
  D5 : Subsystem
  D6 : Subsystem
  D7 : Subsystem
  Ground : powerlib/Elements/Ground  LConnTagsString=a
  Ideal Switch : powerlib/Power Electronics/Ideal Switch  Ron=V^2/(Jug_W+0.000001)  Lon=0  IC=0  Rs=1e5  Cs=inf  Measurements=on
  + : PMIOPort  Side=Left
  wires:
  Add/1 -> Ideal Switch/1
  D1/1(Out1) -> Add/1
  D2/1(Out1) -> Add/2
  D3/1(Out1) -> Add/3
  D4/1(Out1) -> Add/4
  D5/1(Out1) -> Add/5
  D6/1(Out1) -> Add/6
  D7/1(Out1) -> Add/7
  connections:
  Ground/LConn1 -- Ideal Switch/LConn1
  +/RConn1 -- Ideal Switch/RConn1

== system Microgrid_W/House 3 W2/Lamp 1 ==
  Add : Sum  Inputs=+++++++
  D1 : Subsystem
  D2 : Subsystem
  D3 : Subsystem
  D4 : Subsystem
  D5 : Subsystem
  D6 : Subsystem
  D7 : Subsystem
  Ground : powerlib/Elements/Ground  LConnTagsString=a
  Ideal Switch : powerlib/Power Electronics/Ideal Switch  Ron=V^2/(Lamp_1_W+0.000001)  Lon=0  IC=0  Rs=1e5  Cs=inf  Measurements=on
  + : PMIOPort  Side=Left
  wires:
  Add/1 -> Ideal Switch/1
  D7/1(Out1) -> Add/7
  D6/1(Out1) -> Add/6
  D5/1(Out1) -> Add/5
  D4/1(Out1) -> Add/4
  D3/1(Out1) -> Add/3
  D2/1(Out1) -> Add/2
  D1/1(Out1) -> Add/1
  connections:
  +/RConn1 -- Ideal Switch/RConn1
  Ground/LConn1 -- Ideal Switch/LConn1

== system Microgrid_W/House 3 W2/Lamp 2 ==
  Add : Sum  Inputs=+++++++
  D1 : Subsystem
  D2 : Subsystem
  D3 : Subsystem
  D4 : Subsystem
  D5 : Subsystem
  D6 : Subsystem
  D7 : Subsystem
  Ground : powerlib/Elements/Ground  LConnTagsString=a
  Ideal Switch : powerlib/Power Electronics/Ideal Switch  Ron=V^2/(Lamp_2_W+0.000001)  Lon=0  IC=0  Rs=1e5  Cs=inf  Measurements=on
  + : PMIOPort  Side=Left
  wires:
  Add/1 -> Ideal Switch/1
  D1/1(Out1) -> Add/1
  D2/1(Out1) -> Add/2
  D3/1(Out1) -> Add/3
  D4/1(Out1) -> Add/4
  D5/1(Out1) -> Add/5
  D6/1(Out1) -> Add/6
  D7/1(Out1) -> Add/7
  connections:
  +/RConn1 -- Ideal Switch/RConn1
  Ground/LConn1 -- Ideal Switch/LConn1

== system Microgrid_W/House 3 W2/Lamp 3 ==
  Add : Sum  Inputs=+++++++
  D1 : Subsystem
  D2 : Subsystem
  D3 : Subsystem
  D4 : Subsystem
  D5 : Subsystem
  D6 : Subsystem
  D7 : Subsystem
  Ground : powerlib/Elements/Ground  LConnTagsString=a
  Ideal Switch : powerlib/Power Electronics/Ideal Switch  Ron=V^2/(Lamp_3_W+0.000001)  Lon=0  IC=0  Rs=1e5  Cs=inf  Measurements=on
  + : PMIOPort  Side=Left
  wires:
  Add/1 -> Ideal Switch/1
  D7/1(Out1) -> Add/7
  D6/1(Out1) -> Add/6
  D5/1(Out1) -> Add/5
  D4/1(Out1) -> Add/4
  D3/1(Out1) -> Add/3
  D2/1(Out1) -> Add/2
  D1/1(Out1) -> Add/1
  connections:
  +/RConn1 -- Ideal Switch/RConn1
  Ground/LConn1 -- Ideal Switch/LConn1

== system Microgrid_W/House 3 W2/Laptop_Charger ==
  Add : Sum  Inputs=+++++++
  Add1 : Sum  Inputs=+++++++
  D1 : Subsystem
  D10 : Subsystem
  D11 : Subsystem
  D12 : Subsystem
  D13 : Subsystem
  D14 : Subsystem
  D2 : Subsystem
  D3 : Subsystem
  D4 : Subsystem
  D5 : Subsystem
  D6 : Subsystem
  D7 : Subsystem
  D8 : Subsystem
  D9 : Subsystem
  Ground : powerlib/Elements/Ground  LConnTagsString=a
  Ground1 : powerlib/Elements/Ground  LConnTagsString=a
  Ideal Switch : powerlib/Power Electronics/Ideal Switch  Ron=V^2/(Laptop_C_1_W+0.000001)  Lon=0  IC=0  Rs=1e5  Cs=inf  Measurements=on
  Ideal Switch1 : powerlib/Power Electronics/Ideal Switch  Ron=V^2/(Laptop_C_2_W+0.000001)  Lon=0  IC=0  Rs=1e5  Cs=inf  Measurements=on
  + : PMIOPort  Side=Left
  +1 : PMIOPort  Port=2  Side=Right
  wires:
  Add/1 -> Ideal Switch1/1
  Add1/1 -> Ideal Switch/1
  D8/1(Out1) -> Add1/1
  D9/1(Out1) -> Add1/2
  D10/1(Out1) -> Add1/3
  D11/1(Out1) -> Add1/4
  D12/1(Out1) -> Add1/5
  D13/1(Out1) -> Add1/6
  D14/1(Out1) -> Add1/7
  D7/1(Out1) -> Add/7
  D6/1(Out1) -> Add/6
  D5/1(Out1) -> Add/5
  D4/1(Out1) -> Add/4
  D3/1(Out1) -> Add/3
  D2/1(Out1) -> Add/2
  D1/1(Out1) -> Add/1
  connections:
  +1/RConn1 -- Ideal Switch1/RConn1
  Ground1/LConn1 -- Ideal Switch1/LConn1
  +/RConn1 -- Ideal Switch/RConn1
  Ground/LConn1 -- Ideal Switch/LConn1

== system Microgrid_W/House 3 W2/Light 1 ==
  Add : Sum  Inputs=+++++++
  D1 : Subsystem
  D2 : Subsystem
  D3 : Subsystem
  D4 : Subsystem
  D5 : Subsystem
  D6 : Subsystem
  D7 : Subsystem
  Ground : powerlib/Elements/Ground  LConnTagsString=a
  Ideal Switch : powerlib/Power Electronics/Ideal Switch  Ron=V^2/(K_L1_W + 0.000001)  Lon=0  IC=0  Rs=1e5  Cs=inf  Measurements=on
  + : PMIOPort  Side=Left
  wires:
  D7/1(Out1) -> Add/7
  D6/1(Out1) -> Add/6
  D5/1(Out1) -> Add/5
  D4/1(Out1) -> Add/4
  D3/1(Out1) -> Add/3
  D2/1(Out1) -> Add/2
  D1/1(Out1) -> Add/1
  Add/1 -> Ideal Switch/1
  connections:
  Ground/LConn1 -- Ideal Switch/LConn1
  +/RConn1 -- Ideal Switch/RConn1

== system Microgrid_W/House 3 W2/Light 2 ==
  Add : Sum  Inputs=+++++++
  D1 : Subsystem
  D2 : Subsystem
  D3 : Subsystem
  D4 : Subsystem
  D5 : Subsystem
  D6 : Subsystem
  D7 : Subsystem
  Ground : powerlib/Elements/Ground  LConnTagsString=a
  Ideal Switch : powerlib/Power Electronics/Ideal Switch  Ron=V^2/(K_L2_W+0.000001)  Lon=0  IC=0  Rs=1e5  Cs=inf  Measurements=on
  + : PMIOPort  Side=Left
  wires:
  Add/1 -> Ideal Switch/1
  D1/1(Out1) -> Add/1
  D2/1(Out1) -> Add/2
  D3/1(Out1) -> Add/3
  D4/1(Out1) -> Add/4
  D5/1(Out1) -> Add/5
  D6/1(Out1) -> Add/6
  D7/1(Out1) -> Add/7
  connections:
  Ground/LConn1 -- Ideal Switch/LConn1
  +/RConn1 -- Ideal Switch/RConn1

== system Microgrid_W/House 3 W2/Light 3 ==
  Add : Sum  Inputs=+++++++
  D1 : Subsystem
  D2 : Subsystem
  D3 : Subsystem
  D4 : Subsystem
  D5 : Subsystem
  D6 : Subsystem
  D7 : Subsystem
  Ground : powerlib/Elements/Ground  LConnTagsString=a
  Ideal Switch : powerlib/Power Electronics/Ideal Switch  Ron=V^2/(K_L3_W+0.000001)  Lon=0  IC=0  Rs=1e5  Cs=inf  Measurements=on
  + : PMIOPort  Side=Left
  wires:
  Add/1 -> Ideal Switch/1
  D1/1(Out1) -> Add/1
  D2/1(Out1) -> Add/2
  D3/1(Out1) -> Add/3
  D4/1(Out1) -> Add/4
  D5/1(Out1) -> Add/5
  D6/1(Out1) -> Add/6
  D7/1(Out1) -> Add/7
  connections:
  +/RConn1 -- Ideal Switch/RConn1
  Ground/LConn1 -- Ideal Switch/LConn1

== system Microgrid_W/House 3 W2/Light 4 ==
  Add : Sum  Inputs=+++++++
  D1 : Subsystem
  D2 : Subsystem
  D3 : Subsystem
  D4 : Subsystem
  D5 : Subsystem
  D6 : Subsystem
  D7 : Subsystem
  Ground : powerlib/Elements/Ground  LConnTagsString=a
  Ideal Switch : powerlib/Power Electronics/Ideal Switch  Ron=V^2/(K_L4_W+0.000001)  Lon=0  IC=0  Rs=1e5  Cs=inf  Measurements=on
  + : PMIOPort  Side=Left
  wires:
  Add/1 -> Ideal Switch/1
  D1/1(Out1) -> Add/1
  D2/1(Out1) -> Add/2
  D3/1(Out1) -> Add/3
  D4/1(Out1) -> Add/4
  D5/1(Out1) -> Add/5
  D6/1(Out1) -> Add/6
  D7/1(Out1) -> Add/7
  connections:
  +/RConn1 -- Ideal Switch/RConn1
  Ground/LConn1 -- Ideal Switch/LConn1

== system Microgrid_W/House 3 W2/Light 5 ==
  Add : Sum  Inputs=+++++++
  D1 : Subsystem
  D2 : Subsystem
  D3 : Subsystem
  D4 : Subsystem
  D5 : Subsystem
  D6 : Subsystem
  D7 : Subsystem
  Ground : powerlib/Elements/Ground  LConnTagsString=a
  Ideal Switch : powerlib/Power Electronics/Ideal Switch  Ron=V^2/(K_L5_W+0.000001)  Lon=0  IC=0  Rs=1e5  Cs=inf  Measurements=on
  + : PMIOPort  Side=Left
  wires:
  Add/1 -> Ideal Switch/1
  D7/1(Out1) -> Add/7
  D6/1(Out1) -> Add/6
  D5/1(Out1) -> Add/5
  D4/1(Out1) -> Add/4
  D3/1(Out1) -> Add/3
  D2/1(Out1) -> Add/2
  D1/1(Out1) -> Add/1
  connections:
  +/RConn1 -- Ideal Switch/RConn1
  Ground/LConn1 -- Ideal Switch/LConn1

== system Microgrid_W/House 3 W2/Light 6 ==
  Add : Sum  Inputs=+++++++
  D1 : Subsystem
  D2 : Subsystem
  D3 : Subsystem
  D4 : Subsystem
  D5 : Subsystem
  D6 : Subsystem
  D7 : Subsystem
  Ground : powerlib/Elements/Ground  LConnTagsString=a
  Ideal Switch : powerlib/Power Electronics/Ideal Switch  Ron=V^2/(K_L6_W+0.000001)  Lon=0  IC=0  Rs=1e5  Cs=inf  Measurements=on
  + : PMIOPort  Side=Left
  wires:
  Add/1 -> Ideal Switch/1
  D1/1(Out1) -> Add/1
  D2/1(Out1) -> Add/2
  D3/1(Out1) -> Add/3
  D4/1(Out1) -> Add/4
  D5/1(Out1) -> Add/5
  D6/1(Out1) -> Add/6
  D7/1(Out1) -> Add/7
  connections:
  +/RConn1 -- Ideal Switch/RConn1
  Ground/LConn1 -- Ideal Switch/LConn1

== system Microgrid_W/House 3 W2/Oven ==
  Add : Sum  Inputs=+++++++
  D1 : Subsystem
  D2 : Subsystem
  D3 : Subsystem
  D4 : Subsystem
  D5 : Subsystem
  D6 : Subsystem
  D7 : Subsystem
  Ground : powerlib/Elements/Ground  LConnTagsString=a
  Ideal Switch : powerlib/Power Electronics/Ideal Switch  Ron=V^2/(825*N_Elements+0.000001)  Lon=0  IC=0  Rs=1e5  Cs=inf  Measurements=on
  + : PMIOPort  Side=Left
  wires:
  Add/1 -> Ideal Switch/1
  D1/1(Out1) -> Add/1
  D2/1(Out1) -> Add/2
  D3/1(Out1) -> Add/3
  D4/1(Out1) -> Add/4
  D5/1(Out1) -> Add/5
  D6/1(Out1) -> Add/6
  D7/1(Out1) -> Add/7
  connections:
  Ground/LConn1 -- Ideal Switch/LConn1
  +/RConn1 -- Ideal Switch/RConn1

== system Microgrid_W/House 3 W2/Phone_Charger ==
  Add : Sum  Inputs=+++++++
  Add1 : Sum  Inputs=+++++++
  Add2 : Sum  Inputs=+++++++
  D1 : Subsystem
  D10 : Subsystem
  D11 : Subsystem
  D12 : Subsystem
  D13 : Subsystem
  D14 : Subsystem
  D15 : Subsystem
  D16 : Subsystem
  D17 : Subsystem
  D18 : Subsystem
  D19 : Subsystem
  D2 : Subsystem
  D20 : Subsystem
  D21 : Subsystem
  D3 : Subsystem
  D4 : Subsystem
  D5 : Subsystem
  D6 : Subsystem
  D7 : Subsystem
  D8 : Subsystem
  D9 : Subsystem
  Ground : powerlib/Elements/Ground  LConnTagsString=a
  Ideal Switch : powerlib/Power Electronics/Ideal Switch  Ron=V^2/(Phone_C_1_W+0.000001)  Lon=0  IC=0  Rs=1e5  Cs=inf  Measurements=on
  Ideal Switch1 : powerlib/Power Electronics/Ideal Switch  Ron=V^2/(Phone_C_2_W+0.000001)  Lon=0  IC=0  Rs=1e5  Cs=inf  Measurements=on
  Ideal Switch2 : powerlib/Power Electronics/Ideal Switch  Ron=V^2/(Phone_C_3_W+0.000001)  Lon=0  IC=0  Rs=1e5  Cs=inf  Measurements=on
  + : PMIOPort  Side=Left
  +1 : PMIOPort  Port=2  Side=Right
  +2 : PMIOPort  Port=3  Side=Left
  wires:
  Add2/1 -> Ideal Switch2/1
  Add1/1 -> Ideal Switch1/1
  Add/1 -> Ideal Switch/1
  D21/1(Out1) -> Add2/7
  D19/1(Out1) -> Add2/6
  D18/1(Out1) -> Add2/5
  D17/1(Out1) -> Add2/4
  D16/1(Out1) -> Add2/3
  D15/1(Out1) -> Add2/2
  D20/1(Out1) -> Add2/1
  D14/1(Out1) -> Add1/7
  D13/1(Out1) -> Add1/6
  D12/1(Out1) -> Add1/5
  D11/1(Out1) -> Add1/4
  D10/1(Out1) -> Add1/3
  D9/1(Out1) -> Add1/2
  D8/1(Out1) -> Add1/1
  D7/1(Out1) -> Add/7
  D6/1(Out1) -> Add/6
  D5/1(Out1) -> Add/5
  D4/1(Out1) -> Add/4
  D3/1(Out1) -> Add/3
  D2/1(Out1) -> Add/2
  D1/1(Out1) -> Add/1
  connections:
  +2/RConn1 -- Ideal Switch2/RConn1
  +1/RConn1 -- Ideal Switch1/RConn1
  +/RConn1 -- Ideal Switch/RConn1
  Ideal Switch/LConn1 -- Ideal Switch1/LConn1 -- Ideal Switch2/LConn1 -- Ground/LConn1

== system Microgrid_W/House 3 W2/Refrigerator ==
  Current Measurement : powerlib/Measurements/Current Measurement  PhasorSimulation=off  OutputType=Complex  PSBequivalent=0
  Ground : powerlib/Elements/Ground  LConnTagsString=a
  Ideal Switch : powerlib/Power Electronics/Ideal Switch  Ron=0.01  Lon=0  IC=0  Rs=1e5  Cs=inf  Measurements=on
  Ideal Switch1 : powerlib/Power Electronics/Ideal Switch  Ron=0.01  Lon=0  IC=0  Rs=1e5  Cs=inf  Measurements=on
  Monostable : powerlib_meascontrol/Logic/Monostable  EdgeDetect=Rising  PulseDuration=0.1*(60/t)  ic=0  Ts=0
      settings: SourceProductBaseCode=PS
  Product : Product
  Series RLC Branch1 : powerlib/Elements/Series RLC Branch  LConnTagsString=__new0  RConnTagsString=__new0  BranchType=R  Resistance=V^2/(2240-Fridge_W)  Inductance=1e-3  SetiL0=off  InitialCurrent=0  Capacitance=1e-6  Setx0=off  InitialVoltage=0  Measurements=None
  Series RLC Branch2 : powerlib/Elements/Series RLC Branch  LConnTagsString=__new0  RConnTagsString=__new0  BranchType=R  Resistance=V^2/Fridge_W  Inductance=1e-3  SetiL0=off  InitialCurrent=0  Capacitance=1e-6  Setx0=off  InitialVoltage=0  Measurements=None
  Subsystem : Subsystem
  Voltage Measurement : powerlib/Measurements/Voltage Measurement  PhasorSimulation=off  OutputType=Complex  PSBequivalent=0
  + : PMIOPort  Side=Left
  wires:
  Monostable/1 -> Ideal Switch1/1
  Voltage Measurement/1 -> Product/2
  Current Measurement/1 -> Product/1
  Subsystem/1(Out1) -> Monostable/1, Ideal Switch/1
  Product/1 -> Subsystem/1(In1)
  connections:
  Series RLC Branch1/LConn1 -- Ideal Switch1/RConn1
  Ideal Switch/RConn1 -- Current Measurement/LConn1
  +/RConn1 -- Ideal Switch1/LConn1 -- Ideal Switch/LConn1
  Series RLC Branch2/LConn1 -- Voltage Measurement/LConn1 -- Current Measurement/RConn1
  Ground/LConn1 -- Series RLC Branch1/RConn1 -- Series RLC Branch2/RConn1 -- Voltage Measurement/LConn2

== system Microgrid_W/House 3 W2/Shower ==
  Add : Sum  Inputs=+++++++
  D1 : Subsystem
  D2 : Subsystem
  D3 : Subsystem
  D4 : Subsystem
  D5 : Subsystem
  D6 : Subsystem
  D7 : Subsystem
  Divide : Product  Inputs=*/
  Gain : Gain  Gain=1/(60*(60/t))
  Mo : Constant  Value=9
  Product : Product
  Product1 : Product
  Subtract : Sum  Inputs=+-
  Subtract1 : Sum  Inputs=+-
  Tc : Constant  Value=7
  Th : Constant  Value=60
  To : Constant  Value=40
  Out1 : Outport  VectorParamsAs1DForOutWhenUnconnected=off
  wires:
  Add/1 -> Product1/2
  D1/1(Out1) -> Add/1
  D2/1(Out1) -> Add/2
  D3/1(Out1) -> Add/3
  D4/1(Out1) -> Add/4
  D5/1(Out1) -> Add/5
  D6/1(Out1) -> Add/6
  D7/1(Out1) -> Add/7
  Divide/1 -> Product1/1
  Gain/1 -> Out1/1
  Product1/1 -> Gain/1
  Product/1 -> Divide/1
  Mo/1 -> Product/1
  Subtract/1 -> Product/2
  Subtract1/1 -> Divide/2
  Th/1 -> Subtract1/2
  To/1 -> Subtract/2
  Tc/1 -> Subtract/1, Subtract1/1

== system Microgrid_W/House 3 W2/Stereo ==
  Add : Sum  Inputs=+++++++
  D1 : Subsystem
  D2 : Subsystem
  D3 : Subsystem
  D4 : Subsystem
  D5 : Subsystem
  D6 : Subsystem
  D7 : Subsystem
  Ground : powerlib/Elements/Ground  LConnTagsString=a
  Ideal Switch : powerlib/Power Electronics/Ideal Switch  Ron=V^2/((Stereo_W/2)*1.7+0.000001)+V^2/(Stereo_W/2)/2.2  Lon=0  IC=0  Rs=1e5  Cs=inf  Measurements=on
  + : PMIOPort  Side=Left
  wires:
  Add/1 -> Ideal Switch/1
  D1/1(Out1) -> Add/1
  D2/1(Out1) -> Add/2
  D3/1(Out1) -> Add/3
  D4/1(Out1) -> Add/4
  D5/1(Out1) -> Add/5
  D6/1(Out1) -> Add/6
  D7/1(Out1) -> Add/7
  connections:
  +/RConn1 -- Ideal Switch/RConn1
  Ground/LConn1 -- Ideal Switch/LConn1

== system Microgrid_W/House 3 W2/Subsystem ==

== system Microgrid_W/House 3 W2/Subsystem1 ==

== system Microgrid_W/House 3 W2/Subsystem2 ==
